simulink model "tesla_models_dynamics"  (R2017a)
settings: Solver=VariableStepAuto  StartTime=0.0  StopTime=4.2  RelTol=1e-3
libraries: simulink x1
settings Model: Creator=ASHU  LastModifiedBy=ASHU

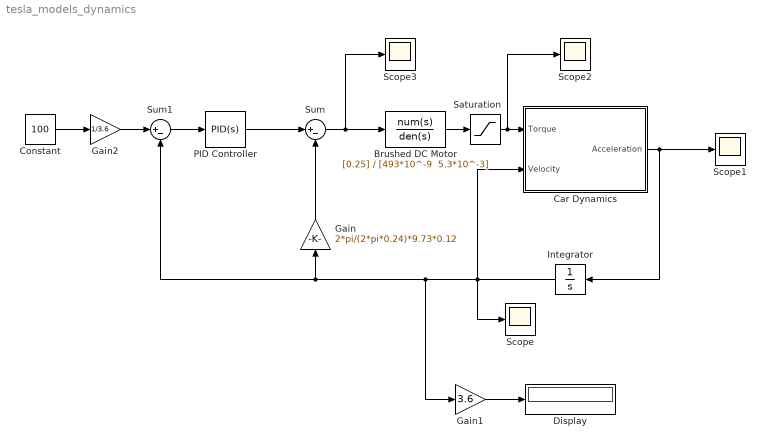
== system tesla_models_dynamics ==
  Brushed DC Motor : TransferFcn  Numerator=[0.25]  Denominator="[493*10^-9  5.3*10^-3]"
  Car Dynamics : MATLAB Function  TreatAsAtomicUnit=on
  Constant : Constant  Value=100
  Display : Display
  Gain : Gain  Gain=2*pi/(2*pi*0.24)*9.73*0.12
  Gain1 : Gain  Gain=3.6
  Gain2 : Gain  Gain=1/3.6
  Integrator : Integrator
  PID Controller : simulink/Continuous/PID Controller  Controller=PID  TimeDomain=Continuous-time  SampleTime=-1  IntegratorMethod=Forward Euler  FilterMethod=Forward Euler  Form=Parallel  UseFilter=on  ControllerParametersSource=internal  P=2000  I=500  D=0  N=100  InitialConditionSource=internal  InitialConditionForIntegrator=0  InitialConditionForFilter=0  ExternalReset=none  LimitOutput=on  UpperSaturationLimit=346  LowerSaturationLimit=0  LinearizeAsGain=on  AntiWindupMode=clamping  Kb=1  TrackingMode=off  Kt=1  PParamMin=[]  PParamMax=[]  IParamMin=[]  IParamMax=[]  DParamMin=[]  DParamMax=[]  NParamMin=[]  NParamMax=[]  KbParamMin=[]  KbParamMax=[]  KtParamMin=[]  KtParamMax=[]  POutMin=[]  POutMax=[]  IOutMin=[]  IOutMax=[]  DOutMin=[]  DOutMax=[]  NOutMin=[]  NOutMax=[]  KbOutMin=[]  KbOutMax=[]  KtOutMin=[]  KtOutMax=[]  IntegratorOutMin=[]  IntegratorOutMax=[]  FilterOutMin=[]  FilterOutMax=[]  SumOutMin=[]  SumOutMax=[]  SumI1OutMin=[]  SumI1OutMax=[]  SumI2OutMin=[]  SumI2OutMax=[]  SumI3OutMin=[]  SumI3OutMax=[]  SumDOutMin=[]  SumDOutMax=[]  SaturationOutMin=[]  SaturationOutMax=[]  IntegratorContinuousStateAttributes=''  IntegratorStateMustResolveToSignalObject=off  IntegratorRTWStateStorageClass=Auto  FilterContinuousStateAttributes=''  FilterStateMustResolveToSignalObject=off  FilterRTWStateStorageClass=Auto  DifferentiatorICPrevScaledInput=0  DifferentiatorOutMin=[]  DifferentiatorOutMax=[]  InitialConditionSetting=State (most efficient)
  Saturation : Saturate  UpperLimit=601  LowerLimit=0
  Scope{,1..3} (4 alike) : Scope
  Sum : Sum  Inputs=|+-
  Sum1 : Sum  Inputs=|+-
  wires:
  Sum/1 -> Scope3/1, Brushed DC Motor/1
  Gain/1 -> Sum/2
  Brushed DC Motor/1 -> Saturation/1
  Car Dynamics/1(Acceleration) -> Scope1/1, Integrator/1
  Integrator/1 -> Scope/1, Gain1/1, Sum1/2, Gain/1, Car Dynamics/2(Velocity)
  Gain1/1 -> Display/1
  Saturation/1 -> Scope2/1, Car Dynamics/1(Torque)
  PID Controller/1 -> Sum/1
  Constant/1 -> Gain2/1
  Gain2/1 -> Sum1/1
  Sum1/1 -> PID Controller/1

== matlab function tesla_models_dynamics/Car Dynamics ==
  data: Torque input; Acceleration output; Velocity input
function Acceleration = fcn(Torque,Velocity)
Acceleration = (40.5*Torque*0.6-413-0.3381*Velocity^2)/2108;
